simulink model "ex_longitudinal_with_vdb"  (R2026a)
settings: Solver=VariableStepAuto
libraries: autolibshared x1
settings Model: Creator=doyeop  LastModifiedBy=doyeop

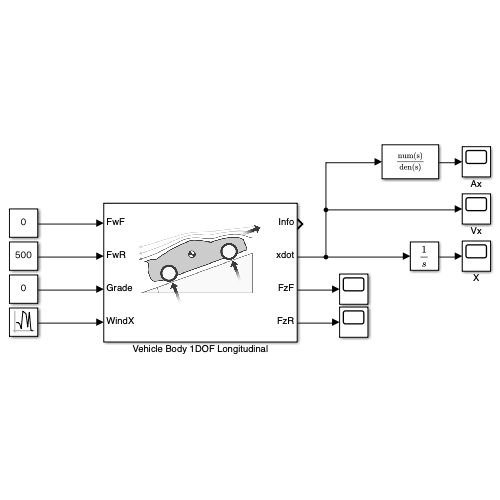
[thumbnail: Simulink's stored preview of the top-level diagram]
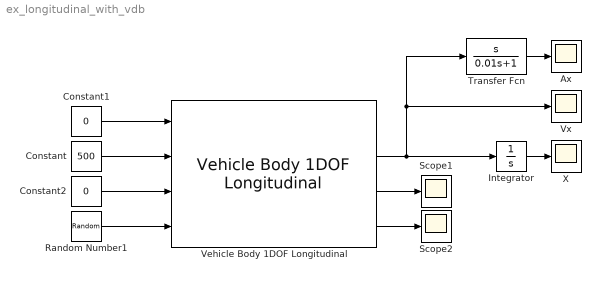
== system ex_longitudinal_with_vdb ==
  Ax : Scope
      settings: ActiveDisplayYMinimum=-0.30908730819720359  ActiveDisplayYMaximum=2.7817857737748328  DataLoggingVariableName=ScopeData3
  Constant : Constant  Value=500
  Constant1 : Constant  Value=0
  Constant2 : Constant  Value=0
  Integrator : Integrator
  Random Number1 : RandomNumber  Mean=3  Variance=0.5^2  SampleTime=0.1
  Scope1 : Scope
      settings: ActiveDisplayYMinimum=237.71250000000009  ActiveDisplayYMaximum=437.71250000000009
  Scope2 : Scope
      settings: ActiveDisplayYMinimum=543.2875  ActiveDisplayYMaximum=743.2875  DataLoggingVariableName=ScopeData2
  Transfer Fcn : TransferFcn  Numerator=[1 0]  Denominator=[0.01 1]
  Vehicle Body 1DOF Longitudinal : autolibshared/Vehicle Body 1DOF Longitudinal  VariantControl=SL  extFMode=off  extMMode=off  extTamb=off  wind3D=off  aMode=1  NF=2  NR=2  m=200  a=1.6*0.6  b=1.6*0.4  h=0.35  Cd=1.0  Cl=0  Cpm=0  Af=0.65  x_o=0  xdot_o=0  Pabs=101325  T=273  g=9.81
      settings: LibrarySourceBlock=autolibvehdynlong/Vehicle Body 1DOF Longitudinal
  Vx : Scope
      settings: ActiveDisplayYMinimum=-2.5143766222464849  ActiveDisplayYMaximum=22.629389600218367
  X : Scope
      settings: ActiveDisplayYMinimum=-13.815713435307774  ActiveDisplayYMaximum=124.34142091777  DataLoggingVariableName=ScopeData4
  wires:
  Constant/1 -> Vehicle Body 1DOF Longitudinal/2
  Vehicle Body 1DOF Longitudinal/2 -> Transfer Fcn/1, Vx/1, Integrator/1
  Constant1/1 -> Vehicle Body 1DOF Longitudinal/1
  Constant2/1 -> Vehicle Body 1DOF Longitudinal/3
  Random Number1/1 -> Vehicle Body 1DOF Longitudinal/4
  Vehicle Body 1DOF Longitudinal/3 -> Scope1/1
  Vehicle Body 1DOF Longitudinal/4 -> Scope2/1
  Transfer Fcn/1 -> Ax/1
  Integrator/1 -> X/1
